simulink model "ACM_RFOC_control_sim"  (R2023a)
settings: Solver=ode23tb  StartTime=0.0  StopTime=100  RelTol=1e-3
values from neighbouring files (symbols this model uses):
  B = 4*0.065*r*tau    (= 0.026)    [ACM_RFOC_control.m]
  eta = 0.95    [ACM_RFOC_control.m]
  J = m*tau^2*r^2    (= 0.8)    [ACM_RFOC_control.m]
  kicdq = 10*100    (= 1000)    [ACM_RFOC_control.m]
  kiw = 2.6*100    (= 260)    [ACM_RFOC_control.m]
  kpcdq = 0.08*100    (= 8)    [ACM_RFOC_control.m]
  kpw = 8*100    (= 800)    [ACM_RFOC_control.m]
  Ld = Ls    (= 0.0008)    [ACM_RFOC_control.m]
  Lq = Ls    (= 0.0008)    [ACM_RFOC_control.m]
  Ls = 0.8e-3    (= 0.0008)    [ACM_RFOC_control.m]
  np = 2    [ACM_RFOC_control.m]
  Pn = 180000    [ACM_RFOC_control.m]
  r = 0.30    (= 0.3)    [ACM_RFOC_control.m]
  Rs = 0.1    [ACM_RFOC_control.m]
  T_braking = [0,T_braking(1),T_braking(1),T_braking(1),T_braking(1),T_braking(1),T_braking(1),T_braking(1),T_braking(1),T_braking(1),T_braking(1),T_braking]*tau    [ACM_RFOC_control.m]
  tau = 1/3    (= 0.333333333333)    [ACM_RFOC_control.m]
  V_bat = 400    [ACM_RFOC_control.m]
  wm_ref = [wm_ref(1),wm_ref(1),wm_ref(1),wm_ref(1),wm_ref(1),wm_ref(1),wm_ref(1),wm_ref(1),wm_ref(1),wm_ref(1),wm_ref]    [ACM_RFOC_control.m]
  Ypm = 0.5    [ACM_RFOC_control.m]
undefined symbols (not defined in the file or in its folder): magnitude
libraries: eeTransforms x10, simulink x6, slpidlib x3, eeSinGeneratorThreePhase x2
settings Model: Creator=Andrea  LastModifiedBy=Andrea
settings DataIOCC: ExternalInput=T_braking  SignalLogging=off  DSMLogging=off

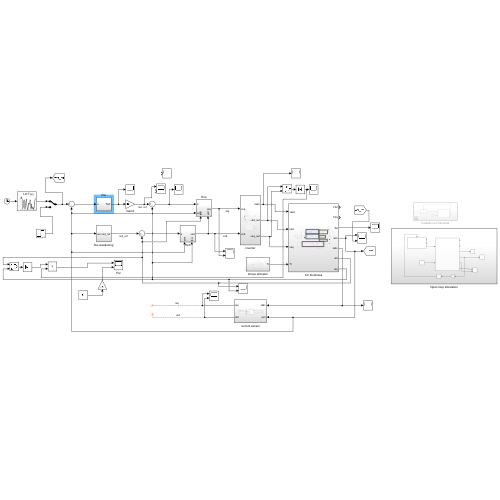
[thumbnail: Simulink's stored preview of the top-level diagram]
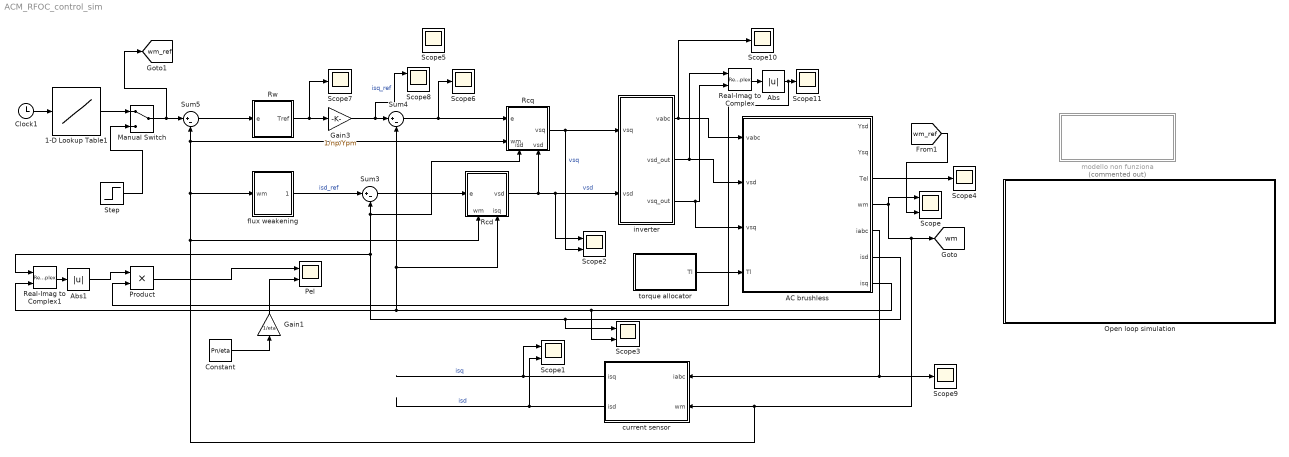
== system ACM_RFOC_control_sim ==
  1-D Lookup Table1 : Lookup_n-D  NumberOfTableDimensions=1  BreakpointsForDimension1=[1:110]  Table=wm_ref  InternalRulePriority=Speed  RndMeth=Simplest
  AC brushless : Subsystem
  Abs : Abs  SaturateOnIntegerOverflow=off
  Abs1 : Abs  SaturateOnIntegerOverflow=off
  Clock1 : Clock
  Constant : Constant  Value=Pn/eta
  Gain1 : Gain  Gain=1/eta
  Gain3 : Gain  Gain=1/np/Ypm
  Manual Switch : ManualSwitch
  Open loop simulation : Subsystem
  Pel : Scope  NumInputPorts=2
  Product : Product
  Rcd : Subsystem
      settings: PortSchema="{\"entries\":[{\"content\":{\"sides\":[{\"content\":{\"connectorIds\":[\"In1\"]},\"type\":\"ConnectorPlacement.EquallySpacedRectSide\",\"uuid\":\"23793d53-caa7-4018-8f4d-565852559395\"},{\"content\":{\"connectorIds\":[\"Out1\"],\"side\":\"RIGHT\"},\"type\":\"ConnectorPlacement.EquallySpacedRectSide\",\"uuid\":\"88f2ca51-1f93-4f76-be8d-3d72c9d34655\"},{\"content\":{\"side\":\"TOP\"},\"type\":\"ConnectorPlacement.EquallySpacedRectSide\",\"uuid\":\"77d93f05-e147-4578-8c10-5fdfccddb555\"},{\"content\":{\"connectorIds\":[\"In2\",\"In3\"],\"side\":\"BOTTOM\"},\"type\":\"ConnectorPlacement.EquallySpacedRectSide\",\"uuid\":\"f8a8ac17-3a4e-4c2c-a5d2-1e0f1c43c6fd\"}]},\"type\":\"ConnectorPlacement.EquallySpacedConnector\",\"uuid\":\"b07d9bbc-e243-43ed-b2c7-1c5a31fa8f78\"}],\"packageUris\":[\"http://schema.mathworks.com/mf0/Connector/R2020b\"],\"version\":\"1.0\"}"
  Rcq : Subsystem
      settings: PortSchema="{\"entries\":[{\"content\":{\"sides\":[{\"content\":{\"connectorIds\":[\"In1\",\"In2\"]},\"type\":\"ConnectorPlacement.EquallySpacedRectSide\",\"uuid\":\"dab87072-766d-41a1-a118-bbd40100a473\"},{\"content\":{\"connectorIds\":[\"Out1\"],\"side\":\"RIGHT\"},\"type\":\"ConnectorPlacement.EquallySpacedRectSide\",\"uuid\":\"2792f500-2696-4550-b610-3ad599a2e919\"},{\"content\":{\"side\":\"TOP\"},\"type\":\"ConnectorPlacement.EquallySpacedRectSide\",\"uuid\":\"5afabe98-fd88-4ded-b895-1d6d2b269472\"},{\"content\":{\"connectorIds\":[\"In3\",\"In4\"],\"side\":\"BOTTOM\"},\"type\":\"ConnectorPlacement.EquallySpacedRectSide\",\"uuid\":\"36dc90c1-3e0f-43e1-9eb1-d8fd404d0fb0\"}]},\"type\":\"ConnectorPlacement.EquallySpacedConnector\",\"uuid\":\"373984ad-aaa1-434b-9efe-1ec2f56933da\"}],\"packageUris\":[\"http://schema.mathworks.com/mf0/Connector/R2020b\"],\"version\":\"1.0\"}"
  Real-Imag to Complex : RealImagToComplex
  Real-Imag to Complex1 : RealImagToComplex
  Rw : Subsystem
  Scope{,1..3,8} (5 alike) : Scope  NumInputPorts=2
  Scope{4..7,9..11} (7 alike) : Scope
  Step : Step  After=2000  SampleTime=0
  Sum3 : Sum  Inputs=|+-
  Sum4 : Sum  Inputs=|+-
  Sum5 : Sum  Inputs=|+-
  current sensor : Subsystem
  flux weakening : Subsystem
  inverter : Subsystem
  modello non funziona : Subsystem  Commented=on
  torque allocator : Subsystem
  tag scope: wm=global, wm_ref=global
  wires:
  inverter/1(vabc) -> Scope10/1, AC brushless/1(vabc)
  AC brushless/5(iabc) -> Scope9/1, current sensor/1(iabc)
  current sensor/2(isd) -> Scope1/2  "isd"
  current sensor/1(isq) -> Scope1/1  "isq"
  AC brushless/4(wm) -> Rcd/2(wm), flux weakening/1(wm), Sum5/2, Rcq/2(wm), current sensor/2(wm), [wm], Scope/1
  Gain3/1 -> Scope8/1, Sum4/1  "isq_ref"
  flux weakening/1(isd_ref) -> Sum3/1  "isd_ref"
  Sum3/1 -> Rcd/1(e)
  Rcd/1(vsd) -> Rcq/4(vsd), Scope2/1, inverter/2(vsd)  "vsd"
  Sum4/1 -> Scope6/1, Rcq/1(e)
  Rcq/1(vsq) -> Scope2/2, inverter/1(vsq)  "vsq"
  Step/1 -> Manual Switch/2
  inverter/2(vsd_out) -> Real-Imag to Complex/1, AC brushless/2(vsd)
  inverter/3(vsq_out) -> Real-Imag to Complex/2, AC brushless/3(vsq)
  AC brushless/3(Tel) -> Scope4/1
  Clock1/1 -> 1-D Lookup Table1/1
  1-D Lookup Table1/1 -> Manual Switch/1
  Manual Switch/1 -> [wm_ref], Sum5/1
  Real-Imag to Complex/1 -> Abs/1
  Abs/1 -> Product/2, Scope11/1
  [wm_ref] -> Scope/2
  Real-Imag to Complex1/1 -> Abs1/1
  AC brushless/7(isq) -> Real-Imag to Complex1/2, Rcd/3(isq), Sum4/2, Scope3/2
  AC brushless/6(isd) -> Scope3/1, Real-Imag to Complex1/1, Rcq/3(isd), Sum3/2
  Abs1/1 -> Product/1
  torque allocator/1(Tl) -> AC brushless/4(Tl)
  Sum5/1 -> Rw/1(e)
  Constant/1 -> Gain1/1
  Rw/1(Tref) -> Scope7/1, Gain3/1
  Product/1 -> Pel/1
  Gain1/1 -> Pel/2

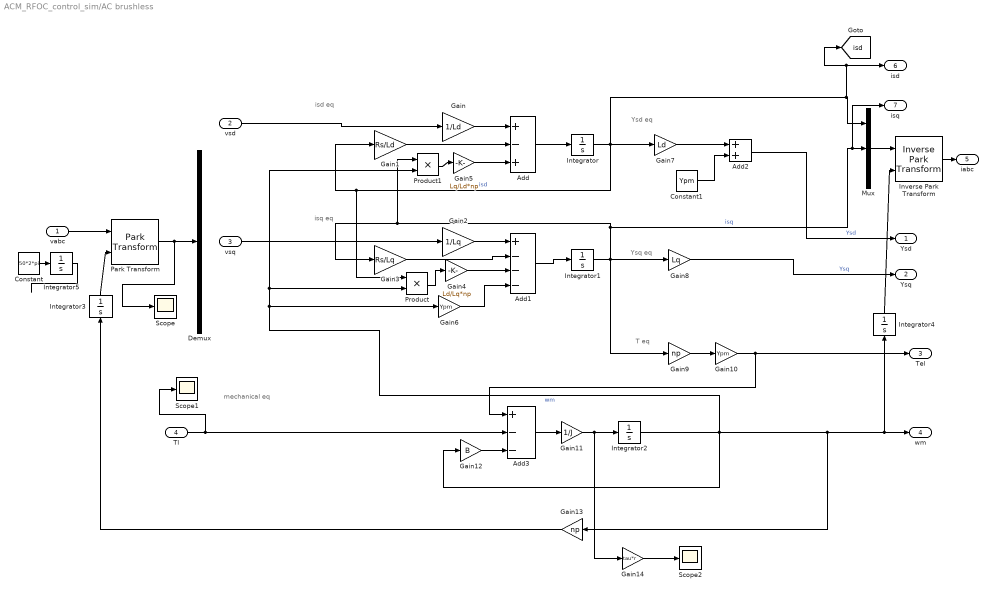
== system ACM_RFOC_control_sim/AC brushless ==
  note: Ysq eq
  note: Ysd eq
  note: isd eq
  note: isq eq
  note: T eq
  note: mechanical eq
  vabc : Inport
  vsd : Inport  Port=2
  vsq : Inport  Port=3
  Tl : Inport  Port=4
  Add : Sum  Inputs=+-+
  Add1 : Sum  Inputs=+---
  Add2 : Sum
  Add3 : Sum  Inputs=+--
  Constant : Constant  Value=50*2*pi
  Constant1 : Constant  Value=Ypm
  Demux : Demux  Outputs=3
  Gain : Gain  Gain=1/Ld
  Gain1 : Gain  Gain=Rs/Ld
  Gain10 : Gain  Gain=Ypm
  Gain11 : Gain  Gain=1/J
  Gain12 : Gain  Gain=B
  Gain13 : Gain  Gain=np
  Gain14 : Gain  Gain=tau*r
  Gain2 : Gain  Gain=1/Lq
  Gain3 : Gain  Gain=Rs/Lq
  Gain4 : Gain  Gain=Ld/Lq*np
  Gain5 : Gain  Gain=Lq/Ld*np
  Gain6 : Gain  Gain=Ypm
  Gain7 : Gain  Gain=Ld
  Gain8 : Gain  Gain=Lq
  Gain9 : Gain  Gain=np
  Integrator{,1..5} (6 alike) : Integrator
  Inverse Park Transform : eeTransforms/Inverse Park Transform  AxisAlignment=Q-axis  PowerInvariant=off
      settings: LibrarySourceBlock=|
      | ee_sl_lib/Mathematical
      | Transforms/Inverse
      | Park Transform
  Mux : Mux  Inputs=3
  Park Transform : eeTransforms/Park Transform  AxisAlignment=D-axis  PowerInvariant=on
      settings: LibrarySourceBlock=|
      | ee_sl_lib/Mathematical
      | Transforms/Park Transform
  Product : Product
  Product1 : Product
  Scope : Scope
  Scope1 : Scope
  Scope2 : Scope
  Ysd : Outport
  Ysq : Outport  Port=2
  Tel : Outport  Port=3
  wm : Outport  Port=4
  iabc : Outport  Port=5
  isd : Outport  Port=6
  isq : Outport  Port=7
  tag scope: isd=global
  wires:
  Integrator4/1 -> Inverse Park Transform/2
  Inverse Park Transform/1 -> iabc/1
  Mux/1 -> Inverse Park Transform/1
  Integrator3/1 -> Park Transform/2
  vabc/1 -> Park Transform/1
  Park Transform/1 -> Scope/1, Demux/1
  vsq/1 -> Gain2/1
  Gain11/1 -> Gain14/1, Integrator2/1
  Gain10/1 -> Add3/1, Tel/1
  Gain9/1 -> Gain10/1
  Product/1 -> Gain4/1
  Add/1 -> Integrator/1
  Product1/1 -> Gain5/1
  Gain1/1 -> Add/2
  vsd/1 -> Gain/1
  Gain7/1 -> Add2/1
  Gain4/1 -> Add1/3
  Add3/1 -> Gain11/1
  Gain12/1 -> Add3/3
  Gain3/1 -> Add1/2
  Gain5/1 -> Add/3
  Tl/1 -> Scope1/1, Add3/2
  Integrator2/1 -> Gain12/1, Integrator4/1, wm/1, Gain13/1, Gain6/1, Product/2, Product1/2  "wm"
  Gain2/1 -> Add1/1
  Add2/1 -> Ysd/1  "Ysd"
  Integrator1/1 -> Gain3/1, Product1/1, isq/1, Mux/2, Gain8/1, Gain9/1  "isq"
  Constant1/1 -> Add2/2
  Add1/1 -> Integrator1/1
  Gain6/1 -> Add1/4
  Gain8/1 -> Ysq/1  "Ysq"
  Gain/1 -> Add/1
  Integrator/1 -> Gain1/1, Product/1, Gain7/1, [isd], isd/1, Mux/1  "isd"
  Gain13/1 -> Integrator3/1
  Constant/1 -> Integrator5/1
  Integrator5/1 -> ?
  Gain14/1 -> Scope2/1

== system ACM_RFOC_control_sim/Open loop simulation ==
  AC brushless : Subsystem
  Constant1 : Constant  Value=0
  Gain : Gain  Gain=np
  Integrator : Integrator
  Scope : Scope  NumInputPorts=2
  Scope5 : Scope
  Scope6 : Scope
  Supplying at Vn2 : Subsystem
      settings: PortSchema="{\"entries\":[{\"content\":{\"sides\":[{\"content\":{},\"type\":\"ConnectorPlacement.EquallySpacedRectSide\",\"uuid\":\"f066e957-29cd-4801-b571-8e93d375f40d\"},{\"content\":{\"connectorIds\":[\"Out1\",\"Out2\",\"Out3\"],\"side\":\"RIGHT\"},\"type\":\"ConnectorPlacement.EquallySpacedRectSide\",\"uuid\":\"f6d6fd36-8f51-42f5-beb4-a76e0ae0fab5\"},{\"content\":{\"connectorIds\":[\"In1\"],\"side\":\"TOP\"},\"type\":\"ConnectorPlacement.EquallySpacedRectSide\",\"uuid\":\"23a8580a-e33c-4630-8f69-2e84ac708083\"}]},\"type\":\"ConnectorPlacement.EquallySpacedConnector\",\"uuid\":\"3ffa5b15-fb1b-445d-9a6f-04c2507fc825\"}],\"packageUris\":[\"http://schema.mathworks.com/mf0/Connector/R2020b\"],\"version\":\"1.0\"}"
  wires:
  AC brushless/6(isdq) -> Scope/1
  Integrator/1 -> Supplying at Vn2/1(th_elec)
  AC brushless/4(wm) -> Gain/1, Scope5/1
  Constant1/1 -> AC brushless/2(Tl)
  AC brushless/3(Tel) -> Scope6/1
  Supplying at Vn2/3(vabc) -> AC brushless/1(vabc)
  AC brushless/5(iabc) -> Scope/2
  Gain/1 -> Integrator/1

== system ACM_RFOC_control_sim/Rcd ==
  e : Inport
  wm : Inport  Port=2
  isq : Inport  Port=3
  Gain : Gain  Gain=np*Ls
  Gain1 : Gain  Gain=kicdq/kpcdq
  Product : Product
  Rcd : slpidlib/PID Controller  Controller=PI  Form=Parallel  TimeDomain=Continuous-time  UseExternalTs=off  SampleTime=-1  IntegratorMethod=Forward Euler  FilterMethod=Forward Euler  ControllerParametersSource=internal  P=kpcdq  I=kicdq  UseKiTs=off  D=0  N=100  UseFilter=on  TunerSelectOption=Transfer Function Based (PID Tuner App)  InitialConditionSource=internal  InitialConditionForIntegrator=0  InitialConditionForFilter=0  DifferentiatorICPrevScaledInput=0  ExternalReset=none  TrackingMode=off  Kt=1  LimitOutput=off  SatLimitsSource=internal  UpperSaturationLimit=inf  LowerSaturationLimit=-inf  LinearizeAsGain=on  AntiWindupMode=none  Kb=1  LimitIntegrator=off  UpperIntegratorSaturationLimit=inf  LowerIntegratorSaturationLimit=-inf  POutMin=[]  POutMax=[]  IOutMin=[]  IOutMax=[]  DOutMin=[]  DOutMax=[]  NOutMin=[]  NOutMax=[]  SumOutMin=[]  SumOutMax=[]  SaturationOutMin=[]  SaturationOutMax=[]  PParamMin=[]  PParamMax=[]  IParamMin=[]  IParamMax=[]  DParamMin=[]  DParamMax=[]  NParamMin=[]  NParamMax=[]  KbParamMin=[]  KbParamMax=[]  KtParamMin=[]  KtParamMax=[]  KbOutMin=[]  KbOutMax=[]  KtOutMin=[]  KtOutMax=[]  IntegratorOutMin=[]  IntegratorOutMax=[]  FilterOutMin=[]  FilterOutMax=[]  SumI1OutMin=[]  SumI1OutMax=[]  SumI2OutMin=[]  SumI2OutMax=[]  SumI3OutMin=[]  SumI3OutMax=[]  SumI4OutMin=[]  SumI4OutMax=[]  SumDOutMin=[]  SumDOutMax=[]  DifferentiatorOutMin=[]  DifferentiatorOutMax=[]  FilterDiffOutCoefMin=[]  FilterDiffOutCoefMax=[]  ReciprocalOutMin=[]  ReciprocalOutMax=[]  SumDenOutMin=[]  SumDenOutMax=[]  SumNumOutMin=[]  SumNumOutMax=[]  DivideOutMin=[]  DivideOutMax=[]  UdiffTsProdOutMin=[]  UdiffTsProdOutMax=[]  NTsProdOutMin=[]  NTsProdOutMax=[]  UintegralTsProdOutMin=[]  UintegralTsProdOutMax=[]  UngainTsProdOutMin=[]  UngainTsProdOutMax=[]  ClampingZeroOutDataTypeStr=Inherit: Inherit via back propagation  ClampingZeroOutMin=[]  ClampingZeroOutMax=[]  FilterDenConstantOutDataTypeStr=Inherit: Inherit via back propagation  FilterDenConstantOutMin=[]  FilterDenConstantOutMax=[]  PCopyOutDataTypeStr=Inherit: Inherit via back propagation  PCopyOutMin=[]  PCopyOutMax=[]  NCopyOutDataTypeStr=Inherit: Inherit via back propagation  NCopyOutMin=[]  NCopyOutMax=[]  IntegratorContinuousStateAttributes=''  IntegratorStateMustResolveToSignalObject=off  IntegratorRTWStateStorageClass=Auto  FilterContinuousStateAttributes=''  FilterStateMustResolveToSignalObject=off  FilterRTWStateStorageClass=Auto  ParallelPVariant=InternalParameters  IdealPVariant=Disabled  IVariant=InternalParameters  DVariant=Disabled  IntegratorVariant=Continuous  SatVariant=Disabled  AWVariant=Passthrough  PCopyVariant=Disabled  TRVariant=Disabled  FdbkBlocksVariant=Forward  IdealPFdbkVariant=Disabled  SatFdbkVariant=Disabled  DerivativeFilterVariant=Disabled  NVariant=Disabled  NCopyVariant=Disabled_SignalSpec  FilterICVariant=Disabled  IntegratorICVariant=InternalICs  ExternalResetVariant=Disabled  TRSumVariant=Passthrough  SumFdbkVariant=Disabled  SumVariant=Sum_PI  TsampFilterVariant=InternalTs  TsampNgainVariant=Passthrough  TsampIntegralVariant=Disabled_SignalSpec  ExternalSaturationOutDataTypeStr=Inherit: Same as second input
  Saturation : Saturate  UpperLimit=V_bat*sqrt(3/2)/2*2  LowerLimit=-V_bat*sqrt(3/2)/2*2
  Scope : Scope  NumInputPorts=2
  Sum : Sum  Inputs=|+-
  Sum1 : Sum  Inputs=|+-
  Sum2 : Sum  Inputs=++|
  vsd : Outport
  wires:
  Sum/1 -> Saturation/1, Sum1/2  "vsd"
  isq/1 -> Product/1
  wm/1 -> Product/2
  Rcd/1 -> Scope/1, Sum/1  "usd"
  Product/1 -> Gain/1
  Gain/1 -> Sum/2, Scope/2
  Sum1/1 -> Gain1/1
  e/1 -> Sum2/2
  Gain1/1 -> Sum2/1
  Sum2/1 -> Rcd/1
  Saturation/1 -> Sum1/1, vsd/1  "vsd"

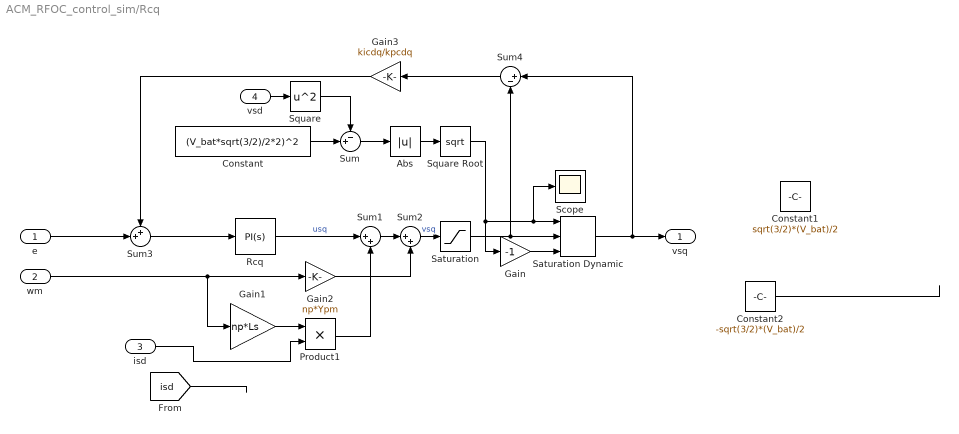
== system ACM_RFOC_control_sim/Rcq ==
  e : Inport
  wm : Inport  Port=2
  isd : Inport  Port=3
  vsd : Inport  Port=4
  Abs : Abs  SaturateOnIntegerOverflow=off
  Constant : Constant  Value=(V_bat*sqrt(3/2)/2*2)^2  VectorParams1D=off
  Constant1 : Constant  Value=sqrt(3/2)*(V_bat)/2
  Constant2 : Constant  Value=-sqrt(3/2)*(V_bat)/2
  Gain : Gain  Gain=-1
  Gain1 : Gain  Gain=np*Ls
  Gain2 : Gain  Gain=np*Ypm
  Gain3 : Gain  Gain=kicdq/kpcdq
  Product1 : Product
  Rcq : slpidlib/PID Controller  Controller=PI  Form=Parallel  TimeDomain=Continuous-time  UseExternalTs=off  SampleTime=-1  IntegratorMethod=Forward Euler  FilterMethod=Forward Euler  ControllerParametersSource=internal  P=kpcdq  I=kicdq  UseKiTs=off  D=0  N=100  UseFilter=on  TunerSelectOption=Transfer Function Based (PID Tuner App)  InitialConditionSource=internal  InitialConditionForIntegrator=0  InitialConditionForFilter=0  DifferentiatorICPrevScaledInput=0  ExternalReset=none  TrackingMode=off  Kt=1  LimitOutput=off  SatLimitsSource=internal  UpperSaturationLimit=inf  LowerSaturationLimit=-inf  LinearizeAsGain=on  AntiWindupMode=none  Kb=1  LimitIntegrator=off  UpperIntegratorSaturationLimit=inf  LowerIntegratorSaturationLimit=-inf  POutMin=[]  POutMax=[]  IOutMin=[]  IOutMax=[]  DOutMin=[]  DOutMax=[]  NOutMin=[]  NOutMax=[]  SumOutMin=[]  SumOutMax=[]  SaturationOutMin=[]  SaturationOutMax=[]  PParamMin=[]  PParamMax=[]  IParamMin=[]  IParamMax=[]  DParamMin=[]  DParamMax=[]  NParamMin=[]  NParamMax=[]  KbParamMin=[]  KbParamMax=[]  KtParamMin=[]  KtParamMax=[]  KbOutMin=[]  KbOutMax=[]  KtOutMin=[]  KtOutMax=[]  IntegratorOutMin=[]  IntegratorOutMax=[]  FilterOutMin=[]  FilterOutMax=[]  SumI1OutMin=[]  SumI1OutMax=[]  SumI2OutMin=[]  SumI2OutMax=[]  SumI3OutMin=[]  SumI3OutMax=[]  SumI4OutMin=[]  SumI4OutMax=[]  SumDOutMin=[]  SumDOutMax=[]  DifferentiatorOutMin=[]  DifferentiatorOutMax=[]  FilterDiffOutCoefMin=[]  FilterDiffOutCoefMax=[]  ReciprocalOutMin=[]  ReciprocalOutMax=[]  SumDenOutMin=[]  SumDenOutMax=[]  SumNumOutMin=[]  SumNumOutMax=[]  DivideOutMin=[]  DivideOutMax=[]  UdiffTsProdOutMin=[]  UdiffTsProdOutMax=[]  NTsProdOutMin=[]  NTsProdOutMax=[]  UintegralTsProdOutMin=[]  UintegralTsProdOutMax=[]  UngainTsProdOutMin=[]  UngainTsProdOutMax=[]  ClampingZeroOutDataTypeStr=Inherit: Inherit via back propagation  ClampingZeroOutMin=[]  ClampingZeroOutMax=[]  FilterDenConstantOutDataTypeStr=Inherit: Inherit via back propagation  FilterDenConstantOutMin=[]  FilterDenConstantOutMax=[]  PCopyOutDataTypeStr=Inherit: Inherit via back propagation  PCopyOutMin=[]  PCopyOutMax=[]  NCopyOutDataTypeStr=Inherit: Inherit via back propagation  NCopyOutMin=[]  NCopyOutMax=[]  IntegratorContinuousStateAttributes=''  IntegratorStateMustResolveToSignalObject=off  IntegratorRTWStateStorageClass=Auto  FilterContinuousStateAttributes=''  FilterStateMustResolveToSignalObject=off  FilterRTWStateStorageClass=Auto  ParallelPVariant=InternalParameters  IdealPVariant=Disabled  IVariant=InternalParameters  DVariant=Disabled  IntegratorVariant=Continuous  SatVariant=Disabled  AWVariant=Passthrough  PCopyVariant=Disabled  TRVariant=Disabled  FdbkBlocksVariant=Forward  IdealPFdbkVariant=Disabled  SatFdbkVariant=Disabled  DerivativeFilterVariant=Disabled  NVariant=Disabled  NCopyVariant=Disabled_SignalSpec  FilterICVariant=Disabled  IntegratorICVariant=InternalICs  ExternalResetVariant=Disabled  TRSumVariant=Passthrough  SumFdbkVariant=Disabled  SumVariant=Sum_PI  TsampFilterVariant=InternalTs  TsampNgainVariant=Passthrough  TsampIntegralVariant=Disabled_SignalSpec  ExternalSaturationOutDataTypeStr=Inherit: Same as second input
  Saturation : Saturate  UpperLimit=V_bat*sqrt(3/2)/2*2-30  LowerLimit=-V_bat*sqrt(3/2)/2*2+30
  Saturation Dynamic : simulink/Discontinuities/Saturation Dynamic  OutMin=[]  OutMax=[]  OutDataTypeStr=Inherit: Same as second input  OutDataType=fixdt(1, 16)  OutScaling=2^-10  DoSatur=off
  Scope : Scope
  Square : Math  Operator=square
  Square Root : Sqrt
  Sum : Sum  Inputs=-+|
  Sum1 : Sum  Inputs=|++
  Sum2 : Sum  Inputs=|++
  Sum3 : Sum  Inputs=++|
  Sum4 : Sum  Inputs=|+-
  vsq : Outport
  wires:
  wm/1 -> Gain2/1, Gain1/1
  Gain1/1 -> Product1/1
  Rcq/1 -> Sum1/1  "usq"
  Gain2/1 -> Sum2/2
  Sum1/1 -> Sum2/1
  [isd] -> ?
  Product1/1 -> Sum1/2
  Saturation Dynamic/1 -> Sum4/1, vsq/1
  vsd/1 -> Square/1
  Constant/1 -> Sum/2
  Sum/1 -> Abs/1
  Square/1 -> Sum/1
  Gain/1 -> Saturation Dynamic/3
  e/1 -> Sum3/2
  Sum3/1 -> Rcq/1
  Sum4/1 -> Gain3/1
  Gain3/1 -> Sum3/1
  isd/1 -> Product1/2
  Square Root/1 -> Scope/1, Saturation Dynamic/1, Gain/1
  Sum2/1 -> Saturation/1  "vsq"
  Saturation/1 -> Saturation Dynamic/2, Sum4/2
  Constant2/1 -> ?
  Abs/1 -> Square Root/1

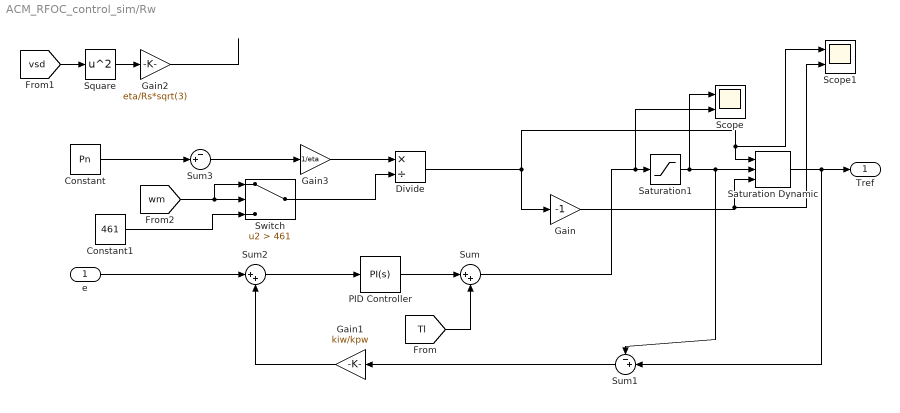
== system ACM_RFOC_control_sim/Rw ==
  e : Inport
  Constant : Constant  Value=Pn
  Constant1 : Constant  Value=461
  Divide : Product  Inputs=*/
  Gain : Gain  Gain=-1
  Gain1 : Gain  Gain=kiw/kpw
  Gain2 : Gain  Gain=eta/Rs*sqrt(3)
  Gain3 : Gain  Gain=1/eta
  PID Controller : slpidlib/PID Controller  Controller=PI  Form=Parallel  TimeDomain=Continuous-time  UseExternalTs=off  SampleTime=-1  IntegratorMethod=Forward Euler  FilterMethod=Forward Euler  ControllerParametersSource=internal  P=kpw  I=kiw  UseKiTs=off  D=0  N=100  UseFilter=on  TunerSelectOption=Transfer Function Based (PID Tuner App)  InitialConditionSource=internal  InitialConditionForIntegrator=0  InitialConditionForFilter=0  DifferentiatorICPrevScaledInput=0  ExternalReset=none  TrackingMode=off  Kt=1  LimitOutput=off  SatLimitsSource=internal  UpperSaturationLimit=1000  LowerSaturationLimit=-1000  LinearizeAsGain=on  AntiWindupMode=back-calculation  Kb=kiw/kpw  LimitIntegrator=off  UpperIntegratorSaturationLimit=inf  LowerIntegratorSaturationLimit=-inf  POutMin=[]  POutMax=[]  IOutMin=[]  IOutMax=[]  DOutMin=[]  DOutMax=[]  NOutMin=[]  NOutMax=[]  SumOutMin=[]  SumOutMax=[]  SaturationOutMin=[]  SaturationOutMax=[]  PParamMin=[]  PParamMax=[]  IParamMin=[]  IParamMax=[]  DParamMin=[]  DParamMax=[]  NParamMin=[]  NParamMax=[]  KbParamMin=[]  KbParamMax=[]  KtParamMin=[]  KtParamMax=[]  KbOutMin=[]  KbOutMax=[]  KtOutMin=[]  KtOutMax=[]  IntegratorOutMin=[]  IntegratorOutMax=[]  FilterOutMin=[]  FilterOutMax=[]  SumI1OutMin=[]  SumI1OutMax=[]  SumI2OutMin=[]  SumI2OutMax=[]  SumI3OutMin=[]  SumI3OutMax=[]  SumI4OutMin=[]  SumI4OutMax=[]  SumDOutMin=[]  SumDOutMax=[]  DifferentiatorOutMin=[]  DifferentiatorOutMax=[]  FilterDiffOutCoefMin=[]  FilterDiffOutCoefMax=[]  ReciprocalOutMin=[]  ReciprocalOutMax=[]  SumDenOutMin=[]  SumDenOutMax=[]  SumNumOutMin=[]  SumNumOutMax=[]  DivideOutMin=[]  DivideOutMax=[]  UdiffTsProdOutMin=[]  UdiffTsProdOutMax=[]  NTsProdOutMin=[]  NTsProdOutMax=[]  UintegralTsProdOutMin=[]  UintegralTsProdOutMax=[]  UngainTsProdOutMin=[]  UngainTsProdOutMax=[]  ClampingZeroOutDataTypeStr=Inherit: Inherit via back propagation  ClampingZeroOutMin=[]  ClampingZeroOutMax=[]  FilterDenConstantOutDataTypeStr=Inherit: Inherit via back propagation  FilterDenConstantOutMin=[]  FilterDenConstantOutMax=[]  PCopyOutDataTypeStr=Inherit: Inherit via back propagation  PCopyOutMin=[]  PCopyOutMax=[]  NCopyOutDataTypeStr=Inherit: Inherit via back propagation  NCopyOutMin=[]  NCopyOutMax=[]  IntegratorContinuousStateAttributes=''  IntegratorStateMustResolveToSignalObject=off  IntegratorRTWStateStorageClass=Auto  FilterContinuousStateAttributes=''  FilterStateMustResolveToSignalObject=off  FilterRTWStateStorageClass=Auto  ParallelPVariant=InternalParameters  IdealPVariant=Disabled  IVariant=InternalParameters  DVariant=Disabled  IntegratorVariant=Continuous  SatVariant=Disabled  AWVariant=Passthrough  PCopyVariant=Disabled  TRVariant=Disabled  FdbkBlocksVariant=Forward  IdealPFdbkVariant=Disabled  SatFdbkVariant=Disabled  DerivativeFilterVariant=Disabled  NVariant=Disabled  NCopyVariant=Disabled_SignalSpec  FilterICVariant=Disabled  IntegratorICVariant=InternalICs  ExternalResetVariant=Disabled  TRSumVariant=Passthrough  SumFdbkVariant=Disabled  SumVariant=Sum_PI  TsampFilterVariant=InternalTs  TsampNgainVariant=Passthrough  TsampIntegralVariant=Disabled_SignalSpec  ExternalSaturationOutDataTypeStr=Inherit: Same as second input
  Saturation Dynamic : simulink/Discontinuities/Saturation Dynamic  OutMin=[]  OutMax=[]  OutDataTypeStr=Inherit: Same as second input  OutDataType=fixdt(1, 16)  OutScaling=2^-10  DoSatur=off
  Saturation1 : Saturate  UpperLimit=Pn-100  LowerLimit=-Pn+100
  Scope : Scope  NumInputPorts=2
  Scope1 : Scope  NumInputPorts=2
  Square : Math  Operator=square
  Sum : Sum  Inputs=|++
  Sum1 : Sum  Inputs=-+|
  Sum2 : Sum  Inputs=|++
  Sum3 : Sum  Inputs=-+|
  Switch : Switch  Criteria=u2 > Threshold  Threshold=461  SaturateOnIntegerOverflow=off  InputSameDT=off
  Tref : Outport
  wires:
  Divide/1 -> Scope1/1, Saturation Dynamic/1, Gain/1
  [Tl] -> Sum/2
  PID Controller/1 -> Sum/1
  [wm] -> Switch/1, Switch/2
  Saturation Dynamic/1 -> Tref/1, Sum1/2
  Sum1/1 -> Gain1/1
  e/1 -> Sum2/1
  Sum2/1 -> PID Controller/1
  Gain1/1 -> Sum2/2
  Sum/1 -> Scope/2, Saturation1/1
  Gain/1 -> Scope1/2, Saturation Dynamic/3
  Saturation1/1 -> Scope/1, Sum1/1, Saturation Dynamic/2
  Constant1/1 -> Switch/3
  Switch/1 -> Divide/2
  Constant/1 -> Sum3/2
  Sum3/1 -> Gain3/1
  [vsd] -> Square/1
  Square/1 -> Gain2/1
  Gain2/1 -> ?
  Gain3/1 -> Divide/1

== system ACM_RFOC_control_sim/current sensor ==
  iabc : Inport
  wm : Inport  Port=2
  Demux : Demux  Outputs=3
  Gain1 : Gain  Gain=np
  Park Transform : eeTransforms/Park Transform  AxisAlignment=D-axis  PowerInvariant=on
      settings: LibrarySourceBlock=|
      | ee_sl_lib/Mathematical
      | Transforms/Park Transform
  isq : Outport
  isd : Outport  Port=2
  wires:
  iabc/1 -> Park Transform/1
  Park Transform/1 -> Demux/1
  Demux/1 -> isd/1
  Demux/2 -> isq/1
  wm/1 -> Gain1/1
  Gain1/1 -> Park Transform/2

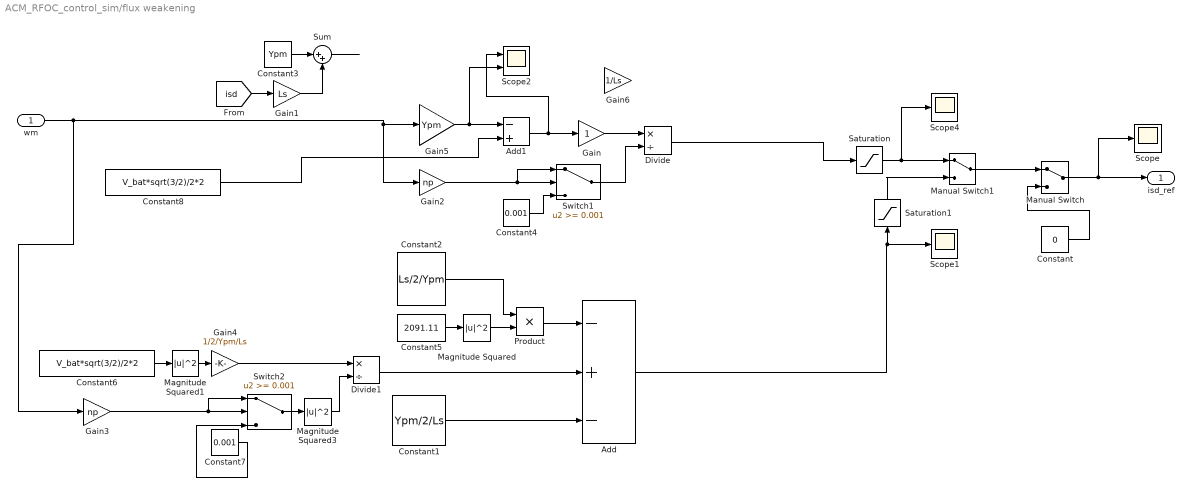
== system ACM_RFOC_control_sim/flux weakening ==
  wm : Inport
  Add : Sum  Inputs=-+-
  Add1 : Sum  Inputs=-+
  Constant : Constant  Value=0
  Constant1 : Constant  Value=Ypm/2/Ls
  Constant2 : Constant  Value=Ls/2/Ypm
  Constant3 : Constant  Value=Ypm
  Constant4 : Constant  Value=0.001
  Constant5 : Constant  Value=2091.11
  Constant6 : Constant  Value=V_bat*sqrt(3/2)/2*2
  Constant7 : Constant  Value=0.001
  Constant8 : Constant  Value=V_bat*sqrt(3/2)/2*2
  Divide : Product  Inputs=*/
  Divide1 : Product  Inputs=*/
  Gain : Gain
  Gain1 : Gain  Gain=Ls
  Gain2 : Gain  Gain=np
  Gain3 : Gain  Gain=np
  Gain4 : Gain  Gain=1/2/Ypm/Ls
  Gain5 : Gain  Gain=Ypm
  Gain6 : Gain  Gain=1/Ls
  Magnitude Squared : Math  Operator=magnitude^2
  Magnitude Squared1 : Math  Operator=magnitude^2
  Magnitude Squared3 : Math  Operator=magnitude^2
  Manual Switch : ManualSwitch
  Manual Switch1 : ManualSwitch
  Product : Product
  Saturation : Saturate  UpperLimit=0  LowerLimit=-1000
  Saturation1 : Saturate  UpperLimit=0  LowerLimit=-1000
  Scope : Scope
  Scope1 : Scope
  Scope2 : Scope  NumInputPorts=2
  Scope4 : Scope
  Sum : Sum  Inputs=|++
  Switch1 : Switch  Threshold=0.001  SaturateOnIntegerOverflow=off  InputSameDT=off
  Switch2 : Switch  Threshold=0.001  SaturateOnIntegerOverflow=off  InputSameDT=off
  isd_ref : Outport
  wires:
  Constant/1 -> Manual Switch/2
  Constant1/1 -> Add/3
  Product/1 -> Add/1
  Constant2/1 -> Product/1
  Gain5/1 -> Scope2/2, Add1/1
  Add1/1 -> Gain/1, Scope2/1
  Gain/1 -> Divide/1
  Switch1/1 -> Divide/2
  Constant4/1 -> Switch1/3
  Constant8/1 -> Add1/2
  Divide/1 -> Saturation/1
  Constant5/1 -> Magnitude Squared/1
  Magnitude Squared/1 -> Product/2
  Constant7/1 -> Switch2/3
  wm/1 -> Gain3/1, Gain2/1, Gain5/1
  Gain4/1 -> Divide1/1
  Constant6/1 -> Magnitude Squared1/1
  Magnitude Squared1/1 -> Gain4/1
  Gain3/1 -> Switch2/1, Switch2/2
  Divide1/1 -> Add/2
  Add/1 -> Scope1/1, Saturation1/1
  Switch2/1 -> Magnitude Squared3/1
  Magnitude Squared3/1 -> Divide1/2
  Manual Switch1/1 -> Manual Switch/1
  Manual Switch/1 -> Scope/1, isd_ref/1
  Saturation/1 -> Scope4/1, Manual Switch1/1
  Gain2/1 -> Switch1/1, Switch1/2
  Saturation1/1 -> Manual Switch1/2
  Sum/1 -> ?
  Constant3/1 -> Sum/1
  [isd] -> Gain1/1
  Gain1/1 -> Sum/2

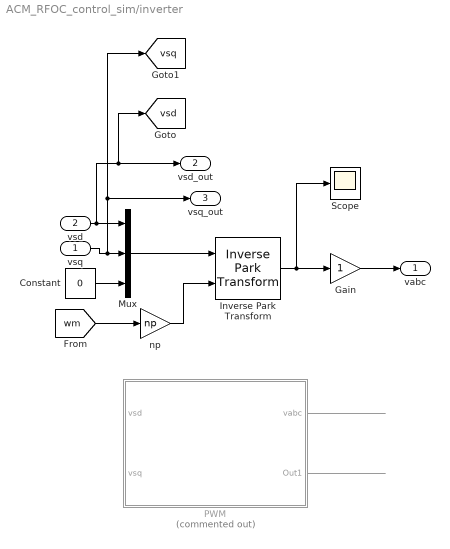
== system ACM_RFOC_control_sim/inverter ==
  vsq : Inport
  vsd : Inport  Port=2
  Constant : Constant  Value=0
  Gain : Gain
  Inverse Park Transform : eeTransforms/Inverse Park Transform  AxisAlignment=D-axis  PowerInvariant=on
      settings: LibrarySourceBlock=|
      | ee_sl_lib/Mathematical
      | Transforms/Inverse
      | Park Transform
  Mux : Mux  Inputs=3
  PWM : Subsystem  Commented=on
  Scope : Scope
  np : Gain  Gain=np
  vabc : Outport
  vsd_out : Outport  Port=2
  vsq_out : Outport  Port=3
  tag scope: vsd=global, vsq=global
  wires:
  vsq/1 -> [vsq], vsq_out/1, Mux/2
  vsd/1 -> [vsd], vsd_out/1, Mux/1
  [wm] -> np/1
  Inverse Park Transform/1 -> Scope/1, Gain/1
  Constant/1 -> Mux/3
  Gain/1 -> vabc/1
  Mux/1 -> Inverse Park Transform/1
  np/1 -> Inverse Park Transform/2
  PWM/1(vabc) -> ?
  PWM/2(Out1) -> ?

== system ACM_RFOC_control_sim/modello non funziona ==
  AC brushless motor (dq) : Subsystem
  Constant : Constant  Value=0
  Supplying at Vn1 : Subsystem
      settings: PortSchema="{\"entries\":[{\"content\":{\"sides\":[{\"content\":{},\"type\":\"ConnectorPlacement.EquallySpacedRectSide\",\"uuid\":\"f066e957-29cd-4801-b571-8e93d375f40d\"},{\"content\":{\"connectorIds\":[\"Out1\"],\"side\":\"RIGHT\"},\"type\":\"ConnectorPlacement.EquallySpacedRectSide\",\"uuid\":\"f6d6fd36-8f51-42f5-beb4-a76e0ae0fab5\"},{\"content\":{\"connectorIds\":[\"In1\"],\"side\":\"TOP\"},\"type\":\"ConnectorPlacement.EquallySpacedRectSide\",\"uuid\":\"23a8580a-e33c-4630-8f69-2e84ac708083\"}]},\"type\":\"ConnectorPlacement.EquallySpacedConnector\",\"uuid\":\"3ffa5b15-fb1b-445d-9a6f-04c2507fc825\"}],\"packageUris\":[\"http://schema.mathworks.com/mf0/Connector/R2020b\"],\"version\":\"1.0\"}"
  wires:
  AC brushless motor (dq)/4(th_elec) -> Supplying at Vn1/1(th_elec)
  Supplying at Vn1/1(dq0) -> AC brushless motor (dq)/1(Vsdq)
  Constant/1 -> AC brushless motor (dq)/2(Tl)

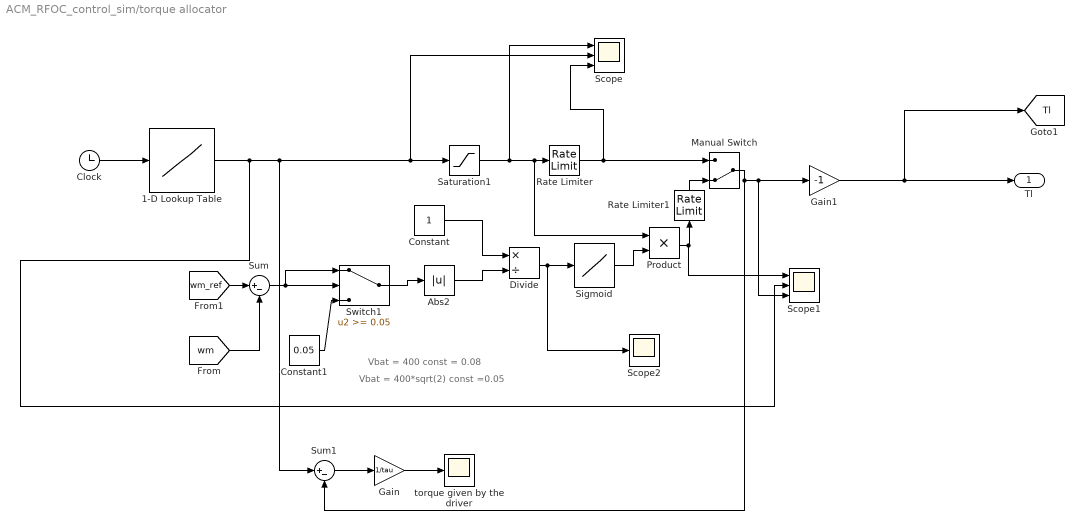
== system ACM_RFOC_control_sim/torque allocator ==
  note: Vbat = 400*sqrt(2) const =0.05
  note: Vbat = 400 const = 0.08
  1-D Lookup Table : Lookup_n-D  NumberOfTableDimensions=1  BreakpointsForDimension1=[1:111]  Table=T_braking  InternalRulePriority=Speed  RndMeth=Simplest
  Abs2 : Abs  SaturateOnIntegerOverflow=off
  Clock : Clock
  Constant : Constant
  Constant1 : Constant  Value=0.05
  Divide : Product  Inputs=*/
  Gain : Gain  Gain=1/tau
  Gain1 : Gain  Gain=-1
  Manual Switch : ManualSwitch  CurrentSetting=0
  Product : Product
  Rate Limiter : RateLimiter  RisingSlewLimit=inf  FallingSlewLimit=-inf  SampleTimeMode=inherited
  Rate Limiter1 : RateLimiter  RisingSlewLimit=1000  FallingSlewLimit=-1000  SampleTimeMode=inherited
  Saturation1 : Saturate  UpperLimit=1000  LowerLimit=-1000
  Scope : Scope  NumInputPorts=3
  Scope1 : Scope  NumInputPorts=3
  Scope2 : Scope
  Sigmoid : Lookup_n-D  NumberOfTableDimensions=1  BreakpointsForDimension1=[0 1 2 3 4 5 6 7 8 9 10]  Table=[4.53978687024459e-05 0.000335350130466483 0.00247262315663477 0.0179862099620915 0.119202922022118 0.5 0.880797077977882 0.982013790037908 0.997527376843365 0.999664649869534 0.999954602131297]  InternalRulePriority=Speed  RndMeth=Simplest
  Sum : Sum  Inputs=|+-
  Sum1 : Sum  Inputs=|+-
  Switch1 : Switch  Threshold=0.05  SaturateOnIntegerOverflow=off  InputSameDT=off
  torque given by the driver : Scope
  Tl : Outport
  tag scope: Tl=global
  wires:
  Saturation1/1 -> Product/1, Rate Limiter/1, Scope/1
  1-D Lookup Table/1 -> Sum1/1, Scope/2, Saturation1/1, Scope1/2
  Clock/1 -> 1-D Lookup Table/1
  [wm_ref] -> Sum/1
  [wm] -> Sum/2
  Manual Switch/1 -> Sum1/2, Scope1/3, Gain1/1
  Rate Limiter/1 -> Manual Switch/1, Scope/3
  Constant/1 -> Divide/1
  Constant1/1 -> Switch1/3
  Product/1 -> Scope1/1, Rate Limiter1/1
  Gain1/1 -> Tl/1, [Tl]
  Sigmoid/1 -> Product/2
  Switch1/1 -> Abs2/1
  Divide/1 -> Scope2/1, Sigmoid/1
  Rate Limiter1/1 -> Manual Switch/2
  Abs2/1 -> Divide/2
  Sum/1 -> Switch1/2, Switch1/1
  Sum1/1 -> Gain/1
  Gain/1 -> torque given by the driver/1

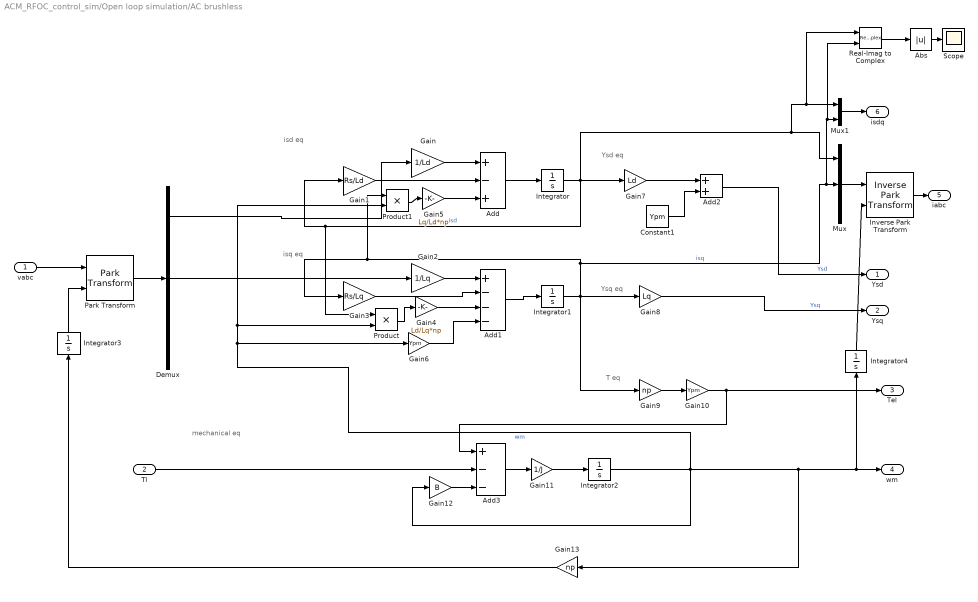
== system ACM_RFOC_control_sim/Open loop simulation/AC brushless ==
  note: mechanical eq
  note: T eq
  note: isq eq
  note: isd eq
  note: Ysd eq
  note: Ysq eq
  vabc : Inport
  Tl : Inport  Port=2
  Abs : Abs  SaturateOnIntegerOverflow=off
  Add : Sum  Inputs=+-+
  Add1 : Sum  Inputs=+---
  Add2 : Sum
  Add3 : Sum  Inputs=+--
  Constant1 : Constant  Value=Ypm
  Demux : Demux  Outputs=3
  Gain : Gain  Gain=1/Ld
  Gain1 : Gain  Gain=Rs/Ld
  Gain10 : Gain  Gain=Ypm
  Gain11 : Gain  Gain=1/J
  Gain12 : Gain  Gain=B
  Gain13 : Gain  Gain=np
  Gain2 : Gain  Gain=1/Lq
  Gain3 : Gain  Gain=Rs/Lq
  Gain4 : Gain  Gain=Ld/Lq*np
  Gain5 : Gain  Gain=Lq/Ld*np
  Gain6 : Gain  Gain=Ypm
  Gain7 : Gain  Gain=Ld
  Gain8 : Gain  Gain=Lq
  Gain9 : Gain  Gain=np
  Integrator{,1..4} (5 alike) : Integrator
  Inverse Park Transform : eeTransforms/Inverse Park Transform  AxisAlignment=Q-axis  PowerInvariant=off
      settings: LibrarySourceBlock=|
      | ee_sl_lib/Mathematical
      | Transforms/Inverse
      | Park Transform
  Mux : Mux  Inputs=3
  Mux1 : Mux  Inputs=2
  Park Transform : eeTransforms/Park Transform  AxisAlignment=D-axis  PowerInvariant=on
      settings: LibrarySourceBlock=|
      | ee_sl_lib/Mathematical
      | Transforms/Park Transform
  Product : Product
  Product1 : Product
  Real-Imag to Complex : RealImagToComplex
  Scope : Scope
  Ysd : Outport
  Ysq : Outport  Port=2
  Tel : Outport  Port=3
  wm : Outport  Port=4
  iabc : Outport  Port=5
  isdq : Outport  Port=6
  wires:
  Integrator/1 -> Real-Imag to Complex/1, Mux1/1, Mux/1, Gain7/1, Product/1, Gain1/1  "isd"
  Gain/1 -> Add/1
  Gain8/1 -> Ysq/1  "Ysq"
  Gain6/1 -> Add1/4
  Add1/1 -> Integrator1/1
  Constant1/1 -> Add2/2
  Integrator1/1 -> Gain9/1, Gain8/1, Real-Imag to Complex/2, Mux1/2, Mux/2, Product1/1, Gain3/1  "isq"
  Add2/1 -> Ysd/1  "Ysd"
  Gain2/1 -> Add1/1
  Integrator2/1 -> Product1/2, Product/2, Gain6/1, Gain13/1, wm/1, Integrator4/1, Gain12/1  "wm"
  Tl/1 -> Add3/2
  Gain5/1 -> Add/3
  Gain3/1 -> Add1/2
  Gain12/1 -> Add3/3
  Add3/1 -> Gain11/1
  Gain4/1 -> Add1/3
  Gain7/1 -> Add2/1
  Demux/1 -> Gain/1
  Gain1/1 -> Add/2
  Product1/1 -> Gain5/1
  Add/1 -> Integrator/1
  Product/1 -> Gain4/1
  Gain9/1 -> Gain10/1
  Gain10/1 -> Tel/1, Add3/1
  Gain11/1 -> Integrator2/1
  Demux/2 -> Gain2/1
  Park Transform/1 -> Demux/1
  vabc/1 -> Park Transform/1
  Integrator3/1 -> Park Transform/2
  Mux/1 -> Inverse Park Transform/1
  Inverse Park Transform/1 -> iabc/1
  Integrator4/1 -> Inverse Park Transform/2
  Mux1/1 -> isdq/1
  Gain13/1 -> Integrator3/1
  Real-Imag to Complex/1 -> Abs/1
  Abs/1 -> Scope/1

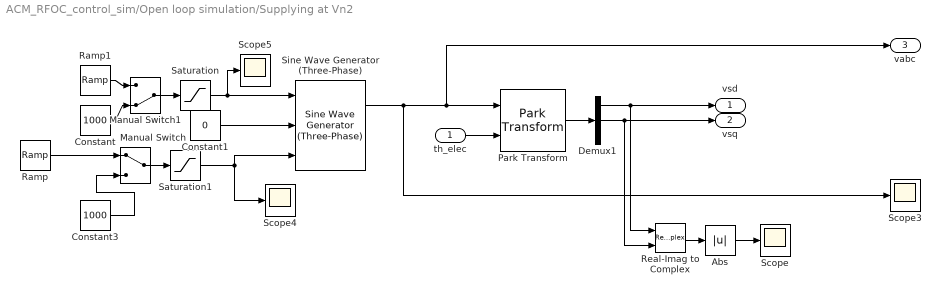
== system ACM_RFOC_control_sim/Open loop simulation/Supplying at Vn2 ==
  th_elec : Inport
  Abs : Abs  SaturateOnIntegerOverflow=off
  Constant : Constant  Value=1000
  Constant1 : Constant  Value=0
  Constant3 : Constant  Value=1000
  Demux1 : Demux  Outputs=3
  Manual Switch : ManualSwitch
  Manual Switch1 : ManualSwitch  CurrentSetting=0
  Park Transform : eeTransforms/Park Transform  AxisAlignment=D-axis  PowerInvariant=on
      settings: LibrarySourceBlock=|
      | ee_sl_lib/Mathematical
      | Transforms/Park Transform
  Ramp : simulink/Sources/Ramp  slope=1  start=0  InitialOutput=0
  Ramp1 : simulink/Sources/Ramp  slope=10  start=0  InitialOutput=0
  Real-Imag to Complex : RealImagToComplex
  Saturation : Saturate  UpperLimit=V_bat*sqrt(1/3)*2  LowerLimit=-V_bat*sqrt(1/3)*2
  Saturation1 : Saturate  UpperLimit=50  LowerLimit=0
  Scope{,3..5} (4 alike) : Scope
  Sine Wave Generator (Three-Phase) : eeSinGeneratorThreePhase/Sine Wave Generator (Three-Phase)  Ts=0
      settings: LibrarySourceBlock=|
      | ee_sl_lib/General Control/Sine Wave Generator
      | (Three-Phase)
  vsd : Outport
  vsq : Outport  Port=2
  vabc : Outport  Port=3
  wires:
  Saturation1/1 -> Sine Wave Generator (Three-Phase)/3, Scope4/1
  Constant1/1 -> Sine Wave Generator (Three-Phase)/2
  Saturation/1 -> Scope5/1, Sine Wave Generator (Three-Phase)/1
  Sine Wave Generator (Three-Phase)/1 -> Scope3/1, vabc/1, Park Transform/1
  Demux1/1 -> Real-Imag to Complex/1, vsd/1
  Demux1/2 -> Real-Imag to Complex/2, vsq/1
  Park Transform/1 -> Demux1/1
  th_elec/1 -> Park Transform/2
  Manual Switch1/1 -> Saturation/1
  Ramp1/1 -> Manual Switch1/1
  Constant/1 -> Manual Switch1/2
  Constant3/1 -> Manual Switch/2
  Manual Switch/1 -> Saturation1/1
  Ramp/1 -> Manual Switch/1
  Real-Imag to Complex/1 -> Abs/1
  Abs/1 -> Scope/1

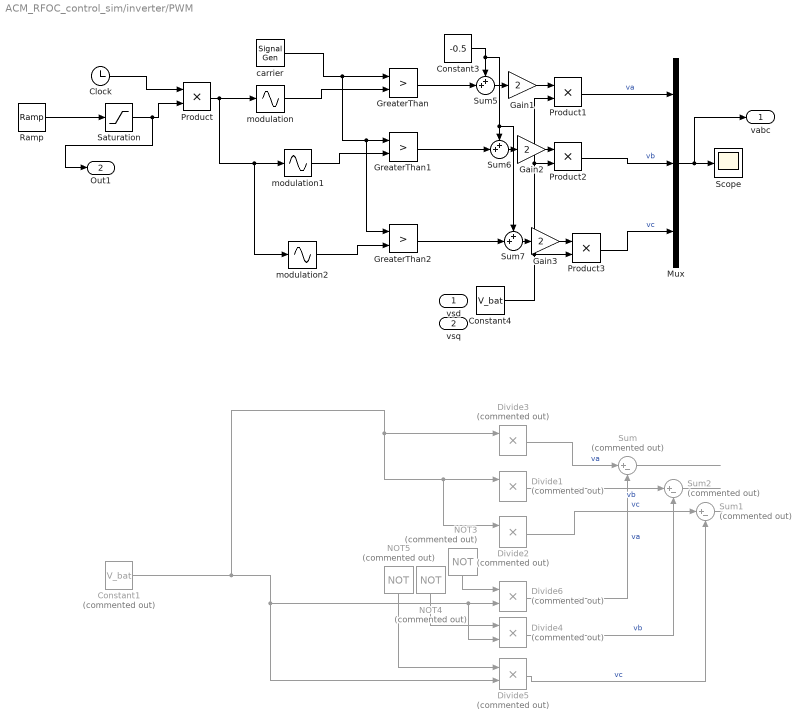
== system ACM_RFOC_control_sim/inverter/PWM ==
  vsd : Inport
  vsq : Inport  Port=2
  Clock : Clock
  Constant1 : Constant  Commented=on  Value=V_bat
  Constant3 : Constant  Value=-0.5
  Constant4 : Constant  Value=V_bat
  Divide{1..6} (6 alike) : Product  Commented=on  Inputs=**
  Gain1 : Gain  Gain=2
  Gain2 : Gain  Gain=2
  Gain3 : Gain  Gain=2
  GreaterThan : RelationalOperator  Operator=>  OutDataTypeStr=boolean  ZeroCross=off  RndMeth=Simplest  InputSameDT=off
  GreaterThan1 : RelationalOperator  Operator=>  OutDataTypeStr=boolean  ZeroCross=off  RndMeth=Simplest  InputSameDT=off
  GreaterThan2 : RelationalOperator  Operator=>  OutDataTypeStr=boolean  ZeroCross=off  RndMeth=Simplest  InputSameDT=off
  Mux : Mux  Inputs=3
  NOT3 : Logic  Commented=on  Operator=NOT  IconShape=distinctive  AllPortsSameDT=off  OutDataTypeStr=boolean
  NOT4 : Logic  Commented=on  Operator=NOT  IconShape=distinctive  AllPortsSameDT=off  OutDataTypeStr=boolean
  NOT5 : Logic  Commented=on  Operator=NOT  IconShape=distinctive  AllPortsSameDT=off  OutDataTypeStr=boolean
  Product{,1..3} (4 alike) : Product
  Ramp : simulink/Sources/Ramp  slope=1  start=0  InitialOutput=0
  Saturation : Saturate  UpperLimit=50*2*pi
  Scope : Scope
  Sum : Sum  Commented=on  Inputs=|+-
  Sum1 : Sum  Commented=on  Inputs=|+-
  Sum2 : Sum  Commented=on  Inputs=|+-
  Sum5 : Sum  Inputs=++|
  Sum6 : Sum  Inputs=++|
  Sum7 : Sum  Inputs=++|
  carrier : SignalGenerator  WaveForm=sawtooth  Frequency=50*pi*2*99  Units=rad/sec
  modulation : Sin  TimeSource=Use external signal  SampleTime=0
  modulation1 : Sin  TimeSource=Use external signal  Phase=-2/3*pi  SampleTime=0
  modulation2 : Sin  TimeSource=Use external signal  Phase=-4/3*pi  SampleTime=0
  vabc : Outport
  Out1 : Outport  Port=2
  wires:
  Sum/1 -> ?
  Divide3/1 -> Sum/1  "va"
  Constant1/1 -> Divide3/1, Divide2/1, Divide1/1, Divide5/2, Divide4/2, Divide6/2
  Sum2/1 -> ?
  Sum1/1 -> ?
  Divide4/1 -> Sum2/2  "vb"
  ? -> NOT5/1, Divide2/2
  ? -> Divide3/2, NOT3/1
  Divide1/1 -> Sum2/1  "vb"
  Divide6/1 -> Sum/2  "va"
  Divide5/1 -> Sum1/2  "vc"
  ? -> NOT4/1, Divide1/2
  NOT4/1 -> Divide4/1
  Divide2/1 -> Sum1/1  "vc"
  NOT3/1 -> Divide6/1
  NOT5/1 -> Divide5/1
  carrier/1 -> GreaterThan2/1, GreaterThan1/1, GreaterThan/1
  modulation/1 -> GreaterThan/2
  Clock/1 -> Product/1
  Ramp/1 -> Saturation/1
  Saturation/1 -> Out1/1, Product/2
  modulation1/1 -> GreaterThan1/2
  Product/1 -> modulation2/1, modulation1/1, modulation/1
  modulation2/1 -> GreaterThan2/2
  Product3/1 -> Mux/3  "vc"
  Constant3/1 -> Sum7/1, Sum6/1, Sum5/1
  Sum7/1 -> Gain3/1
  Constant4/1 -> Product1/2, Product2/2, Product3/2
  Product1/1 -> Mux/1  "va"
  Product2/1 -> Mux/2  "vb"
  Mux/1 -> vabc/1, Scope/1
  GreaterThan/1 -> Sum5/2
  GreaterThan1/1 -> Sum6/2
  GreaterThan2/1 -> Sum7/2
  Sum5/1 -> Gain1/1
  Gain1/1 -> Product1/1
  Sum6/1 -> Gain2/1
  Gain2/1 -> Product2/1
  Gain3/1 -> Product3/1

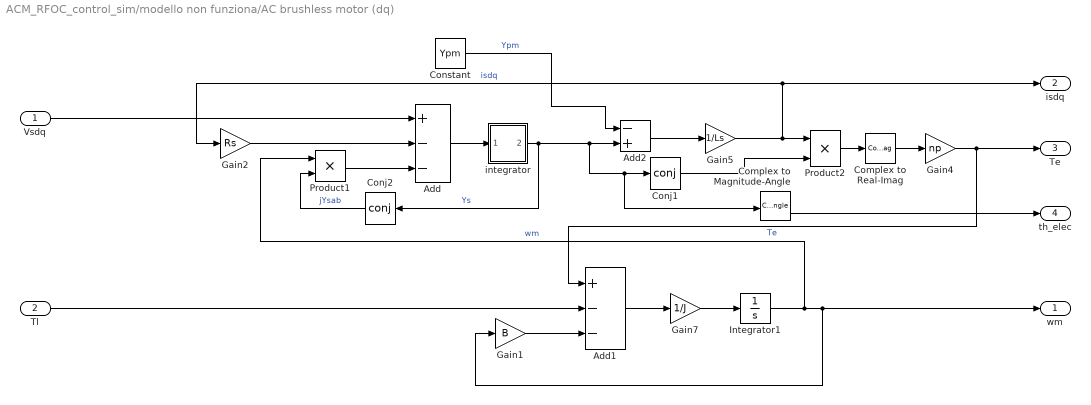
== system ACM_RFOC_control_sim/modello non funziona/AC brushless motor (dq) ==
  Vsdq : Inport
  Tl : Inport  Port=2
  Add : Sum  Inputs=+--
  Add1 : Sum  Inputs=+--
  Add2 : Sum  Inputs=-+
  Complex to Magnitude-Angle : ComplexToMagnitudeAngle
  Complex to Real-Imag : ComplexToRealImag  Output=Imag
  Conj1 : Math  Operator=conj
  Conj2 : Math  Operator=conj
  Constant : Constant  Value=Ypm
  Gain1 : Gain  Gain=B
  Gain2 : Gain  Gain=Rs
  Gain4 : Gain  Gain=np
  Gain5 : Gain  Gain=1/Ls
  Gain7 : Gain  Gain=1/J
  Integrator1 : Integrator
  Product1 : Product
  Product2 : Product
  integrator : Subsystem
  wm : Outport
  isdq : Outport  Port=2
  Te : Outport  Port=3
  th_elec : Outport  Port=4
  wires:
  Product2/1 -> Complex to Real-Imag/1
  Constant/1 -> Add2/1  "Ypm"
  Add/1 -> integrator/1(In1)
  Gain5/1 -> isdq/1, Gain2/1, Product2/1  "isdq"
  Add1/1 -> Gain7/1
  integrator/1(2) -> Conj2/1, Add2/2, Complex to Magnitude-Angle/1, Conj1/1  "Ys"
  Integrator1/1 -> Product1/1, wm/1, Gain1/1  "wm"
  Gain2/1 -> Add/2
  Vsdq/1 -> Add/1
  Add2/1 -> Gain5/1
  Complex to Real-Imag/1 -> Gain4/1
  Gain4/1 -> Te/1, Add1/1  "Te"
  Gain7/1 -> Integrator1/1
  Conj1/1 -> Product2/2
  Gain1/1 -> Add1/3
  Tl/1 -> Add1/2
  Complex to Magnitude-Angle/2 -> th_elec/1
  Product1/1 -> Add/3
  Conj2/1 -> Product1/2  "jYsab"

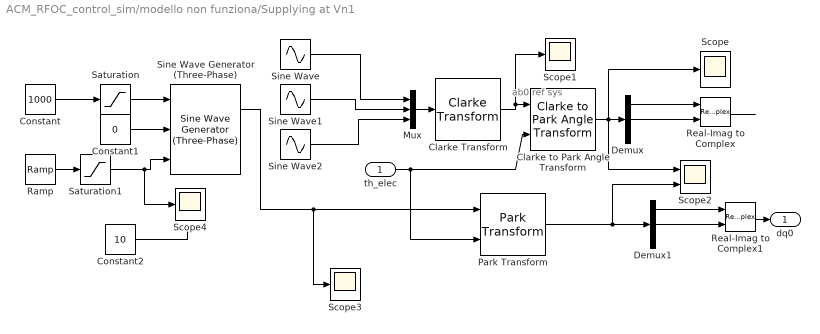
== system ACM_RFOC_control_sim/modello non funziona/Supplying at Vn1 ==
  note: ab0 ref sys
  th_elec : Inport
  Clarke Transform : eeTransforms/Clarke Transform  PowerInvariant=on
      settings: LibrarySourceBlock=|
      | ee_sl_lib/Mathematical
      | Transforms/Clarke Transform
  Clarke to Park Angle Transform : eeTransforms/Clarke to Park Angle Transform  AxisAlignment=D-axis
      settings: LibrarySourceBlock=|
      | ee_sl_lib/Mathematical
      | Transforms/Clarke to Park
      | Angle Transform
  Constant : Constant  Value=1000
  Constant1 : Constant  Value=0
  Constant2 : Constant  Value=10
  Demux : Demux  Outputs=3
  Demux1 : Demux  Outputs=3
  Mux : Mux  Inputs=3
  Park Transform : eeTransforms/Park Transform  AxisAlignment=D-axis  PowerInvariant=on
      settings: LibrarySourceBlock=|
      | ee_sl_lib/Mathematical
      | Transforms/Park Transform
  Ramp : simulink/Sources/Ramp  slope=1  start=0  InitialOutput=0
  Real-Imag to Complex : RealImagToComplex
  Real-Imag to Complex1 : RealImagToComplex
  Saturation : Saturate  UpperLimit=380*sqrt(2)  LowerLimit=-380*sqrt(2)
  Saturation1 : Saturate  UpperLimit=50  LowerLimit=-380*sqrt(2)
  Scope{,1,3..4} (4 alike) : Scope
  Scope2 : Scope  NumInputPorts=2
  Sine Wave : Sin  Frequency=0.01  SampleTime=0
  Sine Wave Generator (Three-Phase) : eeSinGeneratorThreePhase/Sine Wave Generator (Three-Phase)  Ts=0
      settings: LibrarySourceBlock=|
      | ee_sl_lib/General Control/Sine Wave Generator
      | (Three-Phase)
  Sine Wave1 : Sin  Frequency=0.01  Phase=-2/3*pi  SampleTime=0
  Sine Wave2 : Sin  Frequency=0.01  Phase=-4/3*pi  SampleTime=0
  dq0 : Outport
  wires:
  Sine Wave/1 -> Mux/1
  Mux/1 -> Clarke Transform/1
  Sine Wave2/1 -> Mux/3
  Sine Wave1/1 -> Mux/2
  Demux/2 -> Real-Imag to Complex/2
  Demux/1 -> Real-Imag to Complex/1
  Real-Imag to Complex/1 -> ?
  Clarke Transform/1 -> Clarke to Park Angle Transform/1, Scope1/1
  th_elec/1 -> Park Transform/2, Clarke to Park Angle Transform/2
  Clarke to Park Angle Transform/1 -> Scope2/1, Scope/1, Demux/1
  Park Transform/1 -> Scope2/2, Demux1/1
  Demux1/1 -> Real-Imag to Complex1/1
  Demux1/2 -> Real-Imag to Complex1/2
  Real-Imag to Complex1/1 -> dq0/1
  Sine Wave Generator (Three-Phase)/1 -> Scope3/1, Park Transform/1
  Saturation/1 -> Sine Wave Generator (Three-Phase)/1
  Constant1/1 -> Sine Wave Generator (Three-Phase)/2
  Ramp/1 -> Saturation1/1
  Constant2/1 -> ?
  Constant/1 -> Saturation/1
  Saturation1/1 -> Scope4/1, Sine Wave Generator (Three-Phase)/3

== system ACM_RFOC_control_sim/modello non funziona/AC brushless motor (dq)/integrator ==
  note: to avoid numerical issues
  In1 : Inport
  Complex to Real-Imag6 : ComplexToRealImag
  Integrator3 : Integrator
  Integrator4 : Integrator
  Real-Imag to Complex : RealImagToComplex
  2 : Outport
  wires:
  In1/1 -> Complex to Real-Imag6/1
  Complex to Real-Imag6/2 -> Integrator4/1
  Complex to Real-Imag6/1 -> Integrator3/1
  Integrator3/1 -> Real-Imag to Complex/1
  Real-Imag to Complex/1 -> 2/1
  Integrator4/1 -> Real-Imag to Complex/2
